simulink model "float_sch_SigmaDelta_AdaptiveThreshold"  (R2020a)
settings: Solver=VariableStepAuto  StartTime=0  StopTime=1  RelTol=1e-3
values from neighbouring files (symbols this model uses):
  buffer_PWM = 128    [float_sch_run_SigmaDelta_AdaptiveThreshold.m]
  feature_gain = [5]    [float_sch_run_LocalMaxima_AdaptiveThreshold.m]    (also in float_sch_run_Sample_AdaptiveThreshold.m = [7]; float_sch_run_SigmaDelta_AdaptiveThreshold.m)
  fs = 30000    [float_sch_run_LocalMaxima_AdaptiveThreshold.m]    (also in float_sch_run_LocalMaxima_HardThreshold.m; float_sch_run_PTSD.m; float_sch_run_Sample_AdaptiveThreshold.m; float_sch_run_Sample_HardThreshold.m)
  refractory = 10^-3    (= 0.001)    [float_sch_run_LocalMaxima_AdaptiveThreshold.m]    (also in float_sch_run_LocalMaxima_HardThreshold.m; float_sch_run_PTSD.m; float_sch_run_Sample_AdaptiveThreshold.m; float_sch_run_Sample_HardThreshold.m)
  ToStd = 1.27    [float_sch_run_SigmaDelta_AdaptiveThreshold.m]
undefined symbols (not defined in the file or in its folder): DiscIntNeverNeededParam
libraries: dspfdesign x2, dspswit3 x1, simulink x1, hdlsllib x1
settings Model: Creator=diflo  LastModifiedBy=diflo
settings DebuggingCC: SignalRangeChecking=warning

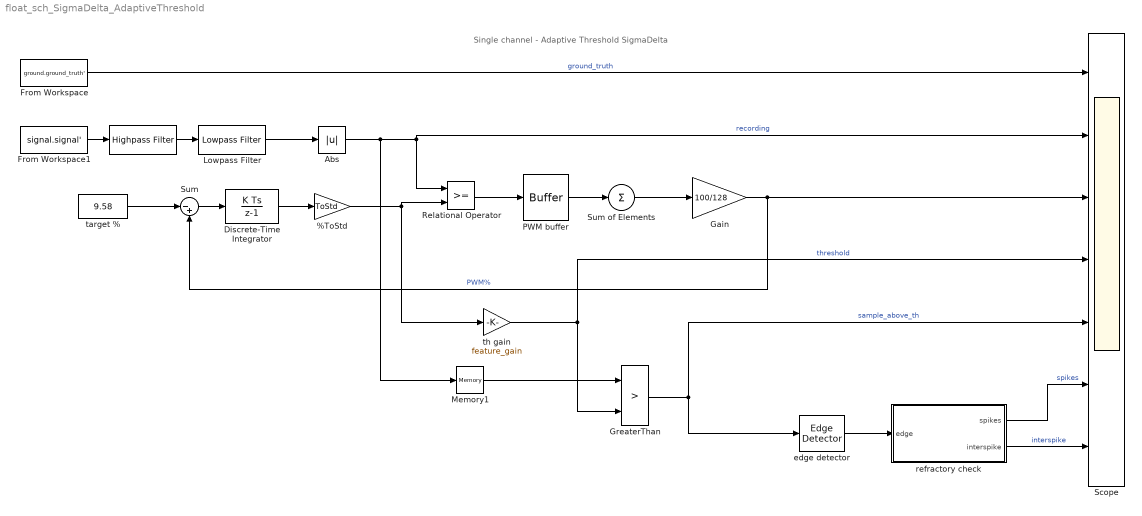
== system float_sch_SigmaDelta_AdaptiveThreshold ==
  note: Single channel - Adaptive Threshold SigmaDelta
  "   " : dspfdesign/Highpass Filter  FilterType=IIR  DesignForMinimumOrder=on  FilterOrder=50  StopbandFrequency=1  PassbandFrequency=300  StopbandAttenuation=80  PassbandRipple=0.1  InheritSampleRate=off  SampleRate=fs  SimulateUsing=Interpreted execution  roundingMode=Floor  coeffsDataTypeStr=fixdt(1,16)
  %ToStd : Gain  Gain=ToStd
  Abs : Abs
  Discrete-Time Integrator : DiscreteIntegrator  gainval=prop_coeff  SampleTime=1/fs  ICPrevOutput=DiscIntNeverNeededParam  ICPrevScaledInput=DiscIntNeverNeededParam
  From Workspace : FromWorkspace  VariableName=ground.ground_truth'  SampleTime=1/fs
  From Workspace1 : FromWorkspace  VariableName=signal.signal'  SampleTime=1/fs
  Gain : Gain  Gain=100/128
  GreaterThan : RelationalOperator  Operator=>  OutDataTypeStr=boolean  RndMeth=Simplest
  Lowpass Filter : dspfdesign/Lowpass Filter  FilterType=IIR  DesignForMinimumOrder=on  FilterOrder=3  PassbandFrequency=3500  StopbandFrequency=8500  PassbandRipple=0.1  StopbandAttenuation=80  InheritSampleRate=off  SampleRate=fs  SimulateUsing=Interpreted execution  roundingMode=Floor  coeffsDataTypeStr=fixdt(1,16)
  Memory1 : Memory  InheritSampleTime=on
  PWM buffer : Buffer  N=buffer_PWM  V=buffer_PWM_overlap  OutputFrames=off
  Relational Operator : RelationalOperator  OutDataTypeStr=boolean
  Scope : Scope  NumInputPorts=7
  Sum : Sum  Inputs=|-+
  Sum of Elements : Sum  Inputs=+
  edge detector : dspswit3/Edge Detector  InputProcessing=Columns as channels (frame based)
      settings: SourceProductBaseCode=DS
  refractory check : Subsystem
  target % : Constant  Value=9.58  SampleTime=1/fs
  th gain : Gain  Gain=feature_gain
  wires:
  Abs/1 -> Memory1/1, Relational Operator/1, Scope/2  "recording"
  target %/1 -> Sum/1
  Relational Operator/1 -> PWM buffer/1
  PWM buffer/1 -> Sum of Elements/1
  Sum of Elements/1 -> Gain/1
  th gain/1 -> Scope/4, GreaterThan/2  "threshold"
  Memory1/1 -> GreaterThan/1
  GreaterThan/1 -> edge detector/1, Scope/5  "sample_above_th"
  Gain/1 -> Sum/2, Scope/3  "PWM%"
  Discrete-Time Integrator/1 -> %ToStd/1
  edge detector/1 -> refractory check/1("  edge ")
  refractory check/1(spikes) -> Scope/6  "spikes"
  refractory check/2(interspike) -> Scope/7  "interspike"
  Sum/1 -> Discrete-Time Integrator/1
  %ToStd/1 -> th gain/1, Relational Operator/2
  From Workspace1/1 -> "   "/1
  From Workspace/1 -> Scope/1  "ground_truth"
  Lowpass Filter/1 -> Abs/1
  "   "/1 -> Lowpass Filter/1

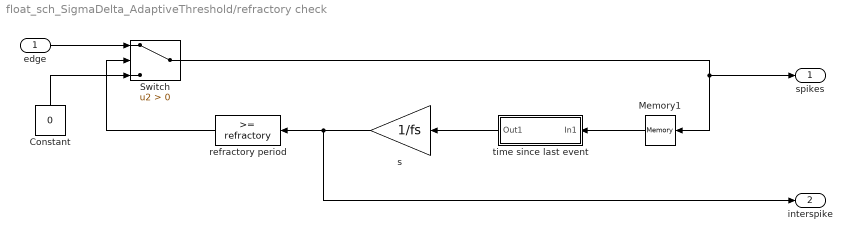
== system float_sch_SigmaDelta_AdaptiveThreshold/refractory check ==
  "  edge " : Inport
  Constant : Constant  Value=0
  Memory1 : Memory  InheritSampleTime=on
  Switch : Switch  Criteria=u2 > Threshold
  refractory period : simulink/Logic and Bit Operations/Compare To Constant  relop=>=  const=refractory  OutDataTypeStr=boolean
  s : Gain  Gain=1/fs  ParamDataTypeStr=double
  time since last event : Subsystem
  spikes : Outport
  interspike : Outport  Port=2
  wires:
  "  edge "/1 -> Switch/1
  Memory1/1 -> time since last event/1(In1)
  time since last event/1(Out1) -> s/1
  Constant/1 -> Switch/3
  s/1 -> refractory period/1, interspike/1
  Switch/1 -> spikes/1, Memory1/1
  refractory period/1 -> Switch/2

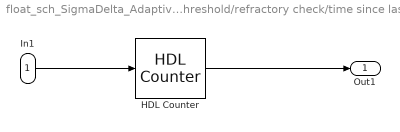
== system float_sch_SigmaDelta_AdaptiveThreshold/refractory check/time since last event ==
  In1 : Inport
  HDL Counter : hdlsllib/Sources/HDL Counter  CountType=Free running  CountInit=1  CountStep=1  CountMax=25  CountFromType=Initial value  CountFrom=1  CountResetPort=on  CountLoadPort=off  CountEnbPort=off  CountDirPort=off  CountDataType=Unsigned  CountWordLen=32  CountFracLen=0  CountSampTime=1
  Out1 : Outport
  wires:
  In1/1 -> HDL Counter/1
  HDL Counter/1 -> Out1/1
